simulink model "sistem_full"  (R2020b)
settings: Solver=ode45  StartTime=0.0  StopTime=10.0  MaxStep=0.01  RelTol=1e-3
undefined symbols (not defined in the file or in its folder): K_d, K_p, params, r_des
(part 1 of 2)
settings Model: Creator=Danil  LastModifiedBy=Danil

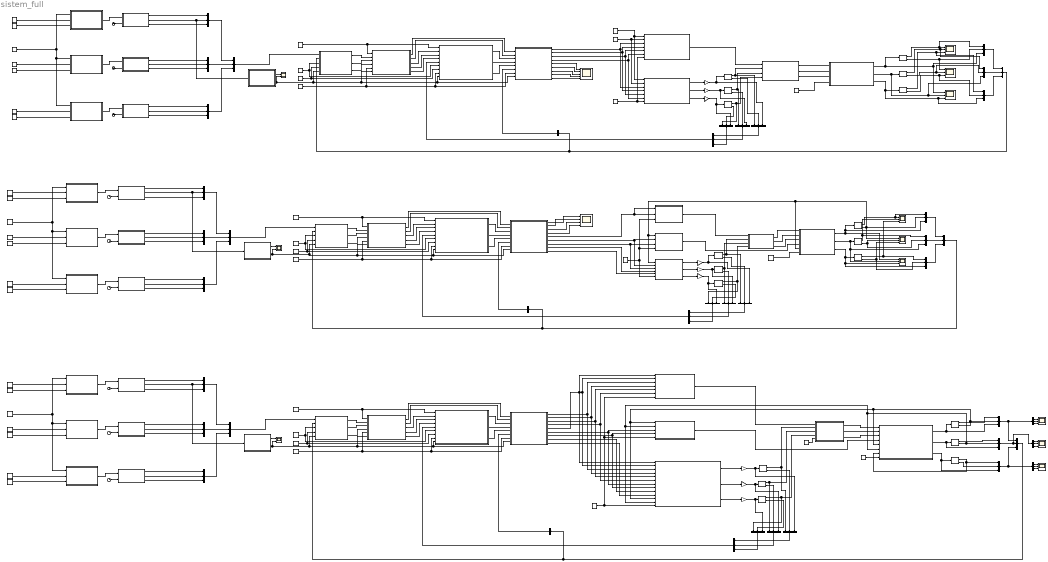
== system sistem_full ==
  note: Координаты X
  note: Траектория движения по оси X
  note: Траектория движения по оси Z
  note: Координаты Z
  note: Траектория движения по оси Y
  note: Координаты Y
  note: Траектория движения по оси Z
  note: Координаты Z
  note: Траектория движения по оси X
  note: Координаты X
  note: Траектория движения по оси Y
  note: Координаты Y
  note: Координаты X
  note: Траектория движения по оси Z
  note: Траектория движения по оси Y
  note: Траектория движения по оси X
  note: Координаты Z
  note: Координаты Y
  Bus Creator{,1..35} (36 alike) : BusCreator  Inputs=3
  Bus Selector : BusSelector  OutputSignals=x.x_dot
  Bus Selector1 : BusSelector  OutputSignals=x.x_dot
  Bus Selector2 : BusSelector  OutputSignals=x,x_dot,x_ddot
  Bus Selector3 : BusSelector  OutputSignals=y,y_dot,y_ddot
  Bus Selector4 : BusSelector  OutputSignals=z,z_dot,z_ddot
  Bus Selector5 : BusSelector  OutputSignals=x.x_dot
  Chart : Stateflow chart  TreatAsAtomicUnit=on
      settings: PortSchema="{\"entries\":[{\"content\":{\"sides\":[{\"content\":{\"connectorIds\":[\"In1\"]},\"type\":\"ConnectorPlacement.EquallySpacedRectSide\",\"uuid\":\"990aaa4d-e872-427e-8bc8-a44f7de52f17\"},{\"content\":{\"connectorIds\":[\"Out2\",\"Out1\"],\"side\":\"RIGHT\"},\"type\":\"ConnectorPlacement.EquallySpacedRectSide\",\"uuid\":\"6e7ad4a8-1d47-4f26-af3c-4dfef899b5bc\"},{\"content\":{\"connectorIds\":[],\"side\":\"TOP\"},\"type\":\"ConnectorPlacement.EquallySpacedRectSide\",\"uuid\":\"20d3b10c-4783-40ca-8243-63709ccaf162\"},{\"content\":{\"connectorIds\":[],\"side\":\"HIDDEN\"},\"type\":\"ConnectorPlacement.EquallySpacedRectSide\",\"uuid\":\"c78cf433-ac9b-47b8-aa1e-24a5718d794b\"}]},\"type\":\"ConnectorPlacement.EquallySpacedConnector\",\"uuid\":\"eb598262-5703-4057-871f-faa738de211a\"}],\"packageUris\":[\"http://schema.mathworks.com/mf0/Connector/R2020b\"],\"version\":\"1.0\"}"
  Chart1 : Stateflow chart  TreatAsAtomicUnit=on
      settings: PortSchema="{\"entries\":[{\"content\":{\"sides\":[{\"content\":{\"connectorIds\":[\"In1\"]},\"type\":\"ConnectorPlacement.EquallySpacedRectSide\",\"uuid\":\"990aaa4d-e872-427e-8bc8-a44f7de52f17\"},{\"content\":{\"connectorIds\":[\"Out2\",\"Out1\"],\"side\":\"RIGHT\"},\"type\":\"ConnectorPlacement.EquallySpacedRectSide\",\"uuid\":\"6e7ad4a8-1d47-4f26-af3c-4dfef899b5bc\"},{\"content\":{\"connectorIds\":[],\"side\":\"TOP\"},\"type\":\"ConnectorPlacement.EquallySpacedRectSide\",\"uuid\":\"20d3b10c-4783-40ca-8243-63709ccaf162\"},{\"content\":{\"connectorIds\":[],\"side\":\"HIDDEN\"},\"type\":\"ConnectorPlacement.EquallySpacedRectSide\",\"uuid\":\"c78cf433-ac9b-47b8-aa1e-24a5718d794b\"}]},\"type\":\"ConnectorPlacement.EquallySpacedConnector\",\"uuid\":\"eb598262-5703-4057-871f-faa738de211a\"}],\"packageUris\":[\"http://schema.mathworks.com/mf0/Connector/R2020b\"],\"version\":\"1.0\"}"
  Chart2 : Stateflow chart  TreatAsAtomicUnit=on
      settings: PortSchema="{\"entries\":[{\"content\":{\"sides\":[{\"content\":{\"connectorIds\":[\"In1\"]},\"type\":\"ConnectorPlacement.EquallySpacedRectSide\",\"uuid\":\"990aaa4d-e872-427e-8bc8-a44f7de52f17\"},{\"content\":{\"connectorIds\":[\"Out2\",\"Out1\"],\"side\":\"RIGHT\"},\"type\":\"ConnectorPlacement.EquallySpacedRectSide\",\"uuid\":\"6e7ad4a8-1d47-4f26-af3c-4dfef899b5bc\"},{\"content\":{\"connectorIds\":[],\"side\":\"TOP\"},\"type\":\"ConnectorPlacement.EquallySpacedRectSide\",\"uuid\":\"20d3b10c-4783-40ca-8243-63709ccaf162\"},{\"content\":{\"connectorIds\":[],\"side\":\"HIDDEN\"},\"type\":\"ConnectorPlacement.EquallySpacedRectSide\",\"uuid\":\"c78cf433-ac9b-47b8-aa1e-24a5718d794b\"}]},\"type\":\"ConnectorPlacement.EquallySpacedConnector\",\"uuid\":\"eb598262-5703-4057-871f-faa738de211a\"}],\"packageUris\":[\"http://schema.mathworks.com/mf0/Connector/R2020b\"],\"version\":\"1.0\"}"
  Clock{,1..8} (9 alike) : Clock
  Constant{,10,13,23..24,26,36} (7 alike) : Constant  Value=params  OutDataTypeStr=Bus: params_bus
  Constant1 : Constant  Value=r_des.x_0
  Constant11 : Constant  Value=0
  Constant12 : Constant  Value=r_des  OutDataTypeStr=Bus: r_des_bus
  Constant14 : Constant  Value=r_des  OutDataTypeStr=Bus: r_des_bus
  Constant15 : Constant  Value=200
  Constant16 : Constant  Value=r_des.time
  Constant17 : Constant  Value=0
  Constant{2,5,18,20} (4 alike) : Constant  Value=2
  Constant19 : Constant  Value=0
  Constant21 : Constant  Value=K_p  OutDataTypeStr=Bus: K_p_bus
  Constant22 : Constant  Value=K_d  OutDataTypeStr=Bus: K_d_bus
  Constant25 : Constant  Value=r_des.x_0
  Constant27 : Constant  Value=r_des  OutDataTypeStr=Bus: r_des_bus
  Constant28 : Constant  Value=r_des.x
  Constant29 : Constant  Value=r_des.time
  Constant3 : Constant  Value=r_des.time
  Constant30 : Constant  Value=r_des.y_0
  Constant31 : Constant  Value=r_des.y
  Constant32 : Constant  Value=r_des.z_0
  Constant33 : Constant  Value=r_des.z
  Constant34 : Constant  Value=K_p  OutDataTypeStr=Bus: K_p_bus
  Constant35 : Constant  Value=K_d  OutDataTypeStr=Bus: K_d_bus
  Constant4 : Constant  Value=r_des.y_0
  Constant6 : Constant  Value=r_des.z_0
  Constant7 : Constant  Value=10
  Constant8 : Constant  Value=K_p  OutDataTypeStr=Bus: K_p_bus
  Constant9 : Constant  Value=K_d  OutDataTypeStr=Bus: K_d_bus
  Gain : Gain  Gain=params.hor.L_x / params.hor.J_xx
  Gain1 : Gain  Gain=params.hor.L_y / params.hor.J_yy
  Gain2 : Gain  Gain=params.hor.L_z / params.hor.J_zz
  Gain3 : Gain  Gain=params.ver.L_x/params.ver.J_xx
  Gain4 : Gain  Gain=params.ver.L_y/params.ver.J_yy
  Gain5 : Gain  Gain=params.ver.L_z/params.ver.J_zz
  Gain6 : Gain  Gain=params.L_x / params.J_xx
  Gain7 : Gain  Gain=params.L_y / params.J_yy
  Gain8 : Gain  Gain=params.L_z / params.J_zz
  Integrator, Second-Order{,1..8,10..17} (17 alike) : SecondOrderIntegrator
  "Integrator, Second-Order9" : SecondOrderIntegrator  ICDXDT=14.1
  MATLAB Function : MATLAB Function  TreatAsAtomicUnit=on
  MATLAB Function1 : MATLAB Function  TreatAsAtomicUnit=on
  MATLAB Function10 : MATLAB Function  TreatAsAtomicUnit=on
  MATLAB Function11 : MATLAB Function  TreatAsAtomicUnit=on
  MATLAB Function12 : MATLAB Function  TreatAsAtomicUnit=on
  MATLAB Function13 : MATLAB Function  TreatAsAtomicUnit=on
  MATLAB Function14 : MATLAB Function  TreatAsAtomicUnit=on
  MATLAB Function15 : MATLAB Function  TreatAsAtomicUnit=on
  MATLAB Function16 : MATLAB Function  TreatAsAtomicUnit=on
  MATLAB Function17 : MATLAB Function  TreatAsAtomicUnit=on
  MATLAB Function18 : MATLAB Function  TreatAsAtomicUnit=on
  MATLAB Function19 : MATLAB Function  TreatAsAtomicUnit=on
  MATLAB Function2 : MATLAB Function  TreatAsAtomicUnit=on
  MATLAB Function20 : MATLAB Function  TreatAsAtomicUnit=on
  MATLAB Function21 : MATLAB Function  TreatAsAtomicUnit=on
  MATLAB Function22 : MATLAB Function  TreatAsAtomicUnit=on
  MATLAB Function23 : MATLAB Function  TreatAsAtomicUnit=on
  MATLAB Function24 : MATLAB Function  TreatAsAtomicUnit=on
  MATLAB Function25 : MATLAB Function  TreatAsAtomicUnit=on
  MATLAB Function26 : MATLAB Function  TreatAsAtomicUnit=on
  MATLAB Function27 : MATLAB Function  TreatAsAtomicUnit=on
  MATLAB Function28 : MATLAB Function  TreatAsAtomicUnit=on
  MATLAB Function29 : MATLAB Function  TreatAsAtomicUnit=on
  MATLAB Function3 : MATLAB Function  TreatAsAtomicUnit=on
  MATLAB Function30 : MATLAB Function  TreatAsAtomicUnit=on
  MATLAB Function31 : MATLAB Function  TreatAsAtomicUnit=on
  MATLAB Function32 : MATLAB Function  TreatAsAtomicUnit=on
  MATLAB Function33 : MATLAB Function  TreatAsAtomicUnit=on
  MATLAB Function34 : MATLAB Function  TreatAsAtomicUnit=on
  MATLAB Function35 : MATLAB Function  TreatAsAtomicUnit=on
  MATLAB Function36 : MATLAB Function  TreatAsAtomicUnit=on
  MATLAB Function37 : MATLAB Function  TreatAsAtomicUnit=on
  MATLAB Function4 : MATLAB Function  TreatAsAtomicUnit=on
  MATLAB Function5 : MATLAB Function  TreatAsAtomicUnit=on
  MATLAB Function6 : MATLAB Function  TreatAsAtomicUnit=on
  MATLAB Function7 : MATLAB Function  TreatAsAtomicUnit=on
  MATLAB Function8 : MATLAB Function  TreatAsAtomicUnit=on
  MATLAB Function9 : MATLAB Function  TreatAsAtomicUnit=on
  Scope{,1..2,5..7,11..13} (9 alike) : Scope  NumInputPorts=3
  Scope10 : Scope  NumInputPorts=2
  Scope3 : Scope  NumInputPorts=2
  Scope4 : Scope  NumInputPorts=5
  Scope8 : Scope  NumInputPorts=2
  Scope9 : Scope  NumInputPorts=4
  Subsystem : Subsystem
  Subsystem1 : Subsystem
  Subsystem2 : Subsystem
  Subsystem3 : Subsystem
  Subsystem4 : Subsystem
  Subsystem5 : Subsystem
  alpha_6 : Constant  Value=params  OutDataTypeStr=Bus: params_bus
  params : Constant  Value=params  OutDataTypeStr=Bus: params_bus
  sigma : Constant  Value=90
  w_L : Constant  Value=params.w_0
  w_R : Constant  Value=params.w_0
  wires:
  Subsystem1/2(M_y) -> MATLAB Function9/4(M_y)
  Subsystem1/3(M_z) -> MATLAB Function9/5(M_z)
  Subsystem/2(y_ddot) -> MATLAB Function7/3(y_ddot)
  Constant8/1 -> Subsystem/3(K_p), Subsystem1/6(K_p)
  Subsystem1/1(M_x) -> MATLAB Function9/3(M_x)
  Chart/1(mode) -> MATLAB Function7/6(mode), MATLAB Function9/8(mode), Subsystem1/9(mode), Subsystem/5(mode), Scope3/2
  MATLAB Function7/4(theta_des) -> Subsystem1/3(theta_des)
  Subsystem/1(x_ddot) -> MATLAB Function7/2(x_ddot)
  Constant10/1 -> MATLAB Function7/5(params), Subsystem1/8(params), MATLAB Function9/7(params)
  MATLAB Function7/1(F_T) -> MATLAB Function9/1(F_T)
  Constant9/1 -> Subsystem/4(K_d), Subsystem1/7(K_d)
  Subsystem/3(z_ddot) -> MATLAB Function7/4(z_ddot)
  MATLAB Function7/5(psi_des) -> Subsystem1/4(psi_des)
  MATLAB Function7/3(fi_des) -> Subsystem1/2(fi_des)
  MATLAB Function7/2(Y) -> MATLAB Function9/2(Y)
  Bus Creator4/1 -> Bus Creator7/1  "x"
  Bus Creator11/1 -> Subsystem1/5(r)
  Bus Creator7/1 -> Bus Selector/1, Subsystem/2(r)
  "Integrator, Second-Order"/2 -> Bus Creator8/2  "fi_dot"
  MATLAB Function11/3(M_z) -> Gain5/1
  "Integrator, Second-Order1"/2 -> Bus Creator9/2  "tehta_dot"
  Bus Creator8/1 -> Bus Creator11/1  "fi"
  "Integrator, Second-Order5"/1 -> Bus Creator6/1, Scope1/3  "z"
  Bus Creator6/1 -> Bus Creator7/3  "z"
  Bus Creator10/1 -> Bus Creator11/3  "psi"
  "Integrator, Second-Order1"/1 -> Bus Creator9/1, MATLAB Function12/3(theta)  "theta"
  Bus Creator9/1 -> Bus Creator11/2  "theta"
  MATLAB Function13/2(y_ddot) -> Bus Creator5/3, Scope2/2, "Integrator, Second-Order4"/1  "y_ddot"
  MATLAB Function9/2(alpha_2) -> MATLAB Function11/4(alpha_2), MATLAB Function10/4(alpha_2)
  "Integrator, Second-Order5"/2 -> Bus Creator6/2, Scope/3  "z_dot"
  Gain3/1 -> Bus Creator8/3, "Integrator, Second-Order"/1  "fi_ddot"
  MATLAB Function12/1(F_x) -> MATLAB Function13/1(F_x)
  MATLAB Function9/4(alpha_4) -> MATLAB Function11/6(alpha_4), MATLAB Function10/6(alpha_4)
  MATLAB Function12/3(F_z) -> MATLAB Function13/3(F_z)
  w_L/1 -> MATLAB Function10/1(w_L), MATLAB Function11/1(w_L)
  MATLAB Function10/1(F) -> MATLAB Function12/1(F)
  Gain5/1 -> "Integrator, Second-Order2"/1, Bus Creator10/3  "psi_ddot"
  alpha_6/1 -> MATLAB Function13/4(params)
  MATLAB Function9/1(alpha_1) -> MATLAB Function11/3(alpha_1), MATLAB Function10/3(alpha_1)
  params/1 -> MATLAB Function10/7(params), MATLAB Function11/7(params)
  MATLAB Function9/3(alpha_3) -> MATLAB Function11/5(alpha_3), MATLAB Function10/5(alpha_3)
  MATLAB Function13/1(x_ddot) -> "Integrator, Second-Order3"/1, Bus Creator4/3, Scope2/1  "x_ddot"
  "Integrator, Second-Order"/1 -> Bus Creator8/1, MATLAB Function12/2(fi)  "fi"
  "Integrator, Second-Order4"/1 -> Bus Creator5/1, Scope1/2  "y"
  "Integrator, Second-Order3"/1 -> Bus Creator4/1, Scope1/1  "x"
  MATLAB Function13/3(z_ddot) -> Bus Creator6/3, Scope2/3, "Integrator, Second-Order5"/1  "z_ddot"
  Gain4/1 -> Bus Creator9/3, "Integrator, Second-Order1"/1  "theta_ddot"
  MATLAB Function11/1(M_x) -> Gain3/1
  "Integrator, Second-Order2"/1 -> Bus Creator10/1, MATLAB Function12/4(psi)  "psi"
  "Integrator, Second-Order4"/2 -> Bus Creator5/2, Scope/2  "y_dot"
  MATLAB Function11/2(M_y) -> Gain4/1
  Bus Creator5/1 -> Bus Creator7/2  "y"
  "Integrator, Second-Order2"/2 -> Bus Creator10/2  "psi_dot"
  MATLAB Function12/2(F_y) -> MATLAB Function13/2(F_y)
  w_R/1 -> MATLAB Function11/2(w_R), MATLAB Function10/2(w_R)
  "Integrator, Second-Order3"/2 -> Bus Creator4/2, Scope/1  "x_dot"
  Constant2/1 -> MATLAB Function5/3(r_end)
  Bus Creator/1 -> Bus Creator3/1  "r_x"
  Bus Creator2/1 -> Bus Creator3/3  "r_z"
  MATLAB Function4/2(vel) -> Chart/1(x_dot_des), Bus Creator/2  "x_dot"
  MATLAB Function2/2(vel) -> Bus Creator2/2  "z_dot"
  Constant7/1 -> MATLAB Function3/3(r_end)
  MATLAB Function/2(vel) -> Bus Creator1/2  "y_dot"
  MATLAB Function/1(pos) -> Bus Creator1/1  "y"
  MATLAB Function1/1(coeff) -> MATLAB Function/1(coeff)
  MATLAB Function2/1(pos) -> Bus Creator2/1  "z"
  Constant6/1 -> MATLAB Function3/2(r_0)
  Constant4/1 -> MATLAB Function1/2(r_0)
  Clock1/1 -> MATLAB Function2/2(clock)
  MATLAB Function3/1(coeff) -> MATLAB Function2/1(coeff)
  Constant3/1 -> MATLAB Function3/1(t), MATLAB Function1/1(t), MATLAB Function5/1(t)
  MATLAB Function5/1(coeff) -> MATLAB Function4/1(coeff)
  Clock/1 -> MATLAB Function/2(clock)
  MATLAB Function4/3(acc) -> Bus Creator/3  "x_ddot"
  Constant5/1 -> MATLAB Function1/3(r_end)
  Constant1/1 -> MATLAB Function5/2(r_0)
  Bus Creator1/1 -> Bus Creator3/2  "r_y"
  MATLAB Function/3(acc) -> Bus Creator1/3  "y_ddot"
  MATLAB Function2/3(acc) -> Bus Creator2/3  "z_ddot"
  Clock2/1 -> MATLAB Function4/2(clock)
  MATLAB Function4/1(pos) -> Bus Creator/1  "x"
  Chart/2(sigma) -> Scope3/1
  MATLAB Function9/9(alpha_F) -> Scope4/5
  MATLAB Function9/5(w) -> Scope4/1
  MATLAB Function9/6(alpha_L) -> Scope4/2
  MATLAB Function9/7(alpha_R) -> Scope4/3
  MATLAB Function9/8(alpha_H) -> Scope4/4
  Bus Selector/1 -> MATLAB Function9/6(x_dot)  "<x_dot>"
  Bus Creator3/1 -> Subsystem/1(r_des)
  Constant12/1 -> MATLAB Function7/1(r_des), Subsystem1/1(r_des)
  Chart1/1(mode) -> MATLAB Function22/6(mode), MATLAB Function23/8(mode), Subsystem3/9(mode), Subsystem2/5(mode), Scope8/2
  Bus Creator17/1 -> Subsystem2/1(r_des)
  MATLAB Function22/2(Y) -> MATLAB Function23/2(Y)
  Clock3/1 -> MATLAB Function6/2(clock)
  MATLAB Function18/3(acc) -> Bus Creator16/3  "z_ddot"
  Clock5/1 -> MATLAB Function20/2(clock)
  MATLAB Function20/3(acc) -> Bus Creator12/3  "x_ddot"
  Subsystem2/1(x_ddot) -> MATLAB Function22/2(x_ddot)
  Chart1/2(sigma) -> Scope8/1
  Subsystem3/3(M_z) -> MATLAB Function23/5(M_z)
  MATLAB Function22/5(psi_des) -> Subsystem3/4(psi_des)
  Constant14/1 -> MATLAB Function22/1(r_des), Subsystem3/1(r_des)
  Constant17/1 -> MATLAB Function8/2(r_0)
  MATLAB Function20/2(vel) -> Chart1/1(x_dot_des), Bus Creator12/2  "x_dot"
  Bus Creator13/1 -> Bus Creator17/2  "r_y"
  Subsystem3/2(M_y) -> MATLAB Function23/4(M_y)
  Constant20/1 -> MATLAB Function19/3(r_end)
  MATLAB Function6/3(acc) -> Bus Creator13/3  "y_ddot"
  Constant16/1 -> MATLAB Function19/1(t), MATLAB Function8/1(t), MATLAB Function21/1(t)
  MATLAB Function20/1(pos) -> Bus Creator12/1  "x"
  Constant18/1 -> MATLAB Function8/3(r_end)
  MATLAB Function6/1(pos) -> Bus Creator13/1  "y"
  MATLAB Function18/2(vel) -> Bus Creator16/2  "z_dot"
  Bus Creator12/1 -> Bus Creator17/1  "r_x"
  MATLAB Function18/1(pos) -> Bus Creator16/1  "z"
  MATLAB Function19/1(coeff) -> MATLAB Function18/1(coeff)
  Constant15/1 -> MATLAB Function21/3(r_end)
  MATLAB Function6/2(vel) -> Bus Creator13/2  "y_dot"
  MATLAB Function8/1(coeff) -> MATLAB Function6/1(coeff)
  MATLAB Function21/1(coeff) -> MATLAB Function20/1(coeff)
  Constant22/1 -> Subsystem2/4(K_d), Subsystem3/7(K_d)
  Constant19/1 -> MATLAB Function19/2(r_0)
  Clock4/1 -> MATLAB Function18/2(clock)
  Subsystem2/3(z_ddot) -> MATLAB Function22/4(z_ddot)
  Bus Creator16/1 -> Bus Creator17/3  "r_z"
  MATLAB Function22/4(theta_des) -> Subsystem3/3(theta_des)
  Constant11/1 -> MATLAB Function21/2(r_0)
  MATLAB Function22/1(F_T) -> MATLAB Function23/1(F_T)
  Constant21/1 -> Subsystem2/3(K_p), Subsystem3/6(K_p)
  Subsystem3/1(M_x) -> MATLAB Function23/3(M_x)
  Constant13/1 -> MATLAB Function22/5(params), Subsystem3/8(params), MATLAB Function23/7(params)
  Subsystem2/2(y_ddot) -> MATLAB Function22/3(y_ddot)
  MATLAB Function22/3(fi_des) -> Subsystem3/2(fi_des)
  Bus Creator19/1 -> Bus Creator21/2  "y"
  MATLAB Function23/6(alpha_L) -> MATLAB Function15/2(alpha_L), MATLAB Function16/2(alpha_L)
  Bus Creator23/1 -> Bus Creator15/2  "theta"
  "Integrator, Second-Order9"/1 -> Bus Creator18/1, Scope6/1  "x"
  Bus Creator15/1 -> Subsystem3/5(r)
  MATLAB Function17/1(F_x) -> MATLAB Function24/1(F_x)
  Bus Creator20/1 -> Bus Creator21/3  "z"
  "Integrator, Second-Order8"/2 -> Bus Creator14/2  "psi_dot"
  "Integrator, Second-Order6"/2 -> Bus Creator22/2  "fi_dot"
  Gain/1 -> Bus Creator22/3, "Integrator, Second-Order6"/1  "fi_ddot"
  Bus Creator21/1 -> Bus Selector1/1, Subsystem2/2(r)
  MATLAB Function16/1(M_x) -> Gain/1
  MATLAB Function24/2(y_ddot) -> Bus Creator19/3, Scope7/2, "Integrator, Second-Order10"/1  "y_ddot"
  Constant24/1 -> MATLAB Function24/6(params)
  "Integrator, Second-Order11"/2 -> Scope5/3, Bus Creator20/2  "z_dot"
  MATLAB Function17/2(F_y) -> MATLAB Function24/2(F_y)
  "Integrator, Second-Order7"/1 -> MATLAB Function17/3(theta), Bus Creator23/1  "theta"
  "Integrator, Second-Order8"/1 -> MATLAB Function17/4(psi), Bus Creator14/1  "psi"
  "Integrator, Second-Order11"/1 -> Bus Creator20/1, Scope6/3  "z"
  MATLAB Function14/1(F) -> MATLAB Function17/1(F)
  Gain1/1 -> Bus Creator23/3, "Integrator, Second-Order7"/1  "theta_ddot"
  Gain2/1 -> Bus Creator14/3, "Integrator, Second-Order8"/1  "psi_ddot"
  "Integrator, Second-Order6"/1 -> Bus Creator22/1, MATLAB Function17/2(fi)  "fi"
  Bus Creator18/1 -> Bus Creator21/1  "x"
  MATLAB Function16/3(M_z) -> Gain2/1
  "Integrator, Second-Order10"/1 -> Bus Creator19/1, Scope6/2  "y"
  MATLAB Function23/8(alpha_H) -> MATLAB Function16/4(alpha_H)
  MATLAB Function17/3(F_z) -> MATLAB Function24/3(F_z)
  MATLAB Function24/1(x_ddot) -> Bus Creator18/3, "Integrator, Second-Order9"/1, Scope7/1  "x_ddot"
  "Integrator, Second-Order10"/2 -> Scope5/2, Bus Creator19/2  "y_dot"
  MATLAB Function23/9(alpha_F) -> MATLAB Function16/5(alpha_F)
  MATLAB Function15/1(Y) -> MATLAB Function24/4(Y)
  MATLAB Function16/2(M_y) -> Gain1/1
  MATLAB Function24/3(z_ddot) -> Bus Creator20/3, Scope7/3, "Integrator, Second-Order11"/1  "z_ddot"
  "Integrator, Second-Order9"/2 -> MATLAB Function24/5(x_dot), MATLAB Function16/1(x_dot), MATLAB Function15/1(x_dot), Bus Creator18/2, Scope5/1  "x_dot"
  Bus Creator22/1 -> Bus Creator15/1  "fi"
  MATLAB Function23/5(w) -> MATLAB Function14/1(w_L), MATLAB Function14/2(w_R)
  Constant23/1 -> MATLAB Function16/6(params), MATLAB Function14/3(params), MATLAB Function15/4(params)
  MATLAB Function23/7(alpha_R) -> MATLAB Function16/3(alpha_R), MATLAB Function15/3(alpha_R)
  "Integrator, Second-Order7"/2 -> Bus Creator23/2  "theta_dot"
  Bus Creator14/1 -> Bus Creator15/3  "psi"
  Bus Selector1/1 -> MATLAB Function23/6(x_dot)  "<x_dot>"
  MATLAB Function23/1(alpha_1) -> Scope9/1
  MATLAB Function23/2(alpha_2) -> Scope9/2
  MATLAB Function23/3(alpha_3) -> Scope9/3
  MATLAB Function23/4(alpha_4) -> Scope9/4
  MATLAB Function26/1(coeff) -> MATLAB Function25/1(coeff)
  Constant31/1 -> MATLAB Function32/3(r_end)
  MATLAB Function29/5(psi_des) -> Subsystem5/4(psi_des)
  Constant27/1 -> MATLAB Function29/1(r_des), Subsystem5/1(r_des)
  MATLAB Function27/3(acc) -> Bus Creator24/3  "x_ddot"
  Bus Creator26/1 -> Bus Creator27/3  "r_z"
  Constant35/1 -> Subsystem4/4(K_d), Subsystem5/7(K_d)
  MATLAB Function27/1(pos) -> Bus Creator24/1  "x"
  MATLAB Function29/3(fi_des) -> Subsystem5/2(fi_des)
  MATLAB Function27/2(vel) -> Chart2/1(x_dot_des), Bus Creator24/2  "x_dot"
  Constant32/1 -> MATLAB Function26/2(r_0)
  Clock7/1 -> MATLAB Function25/2(clock)
  Constant34/1 -> Subsystem4/3(K_p), Subsystem5/6(K_p)
  MATLAB Function28/1(coeff) -> MATLAB Function27/1(coeff)
  Subsystem5/1(M_x) -> MATLAB Function30/3(M_x)
  Subsystem4/2(y_ddot) -> MATLAB Function29/3(y_ddot)
  Chart2/1(mode) -> MATLAB Function29/6(mode), MATLAB Function30/8(mode), Subsystem5/9(mode), Subsystem4/5(mode), Scope10/2
  Subsystem4/1(x_ddot) -> MATLAB Function29/2(x_ddot)
  MATLAB Function29/4(theta_des) -> Subsystem5/3(theta_des)
  Constant25/1 -> MATLAB Function28/2(r_0)
  MATLAB Function29/1(F_T) -> MATLAB Function30/1(F_T)
  Subsystem4/3(z_ddot) -> MATLAB Function29/4(z_ddot)
  MATLAB Function31/1(pos) -> Bus Creator25/1  "y"
  MATLAB Function31/3(acc) -> Bus Creator25/3  "y_ddot"
  MATLAB Function31/2(vel) -> Bus Creator25/2  "y_dot"
  Constant28/1 -> MATLAB Function28/3(r_end)
  MATLAB Function25/1(pos) -> Bus Creator26/1  "z"
  Bus Creator24/1 -> Bus Creator27/1  "r_x"
  MATLAB Function32/1(coeff) -> MATLAB Function31/1(coeff)
  MATLAB Function25/2(vel) -> Bus Creator26/2  "z_dot"
  Subsystem5/3(M_z) -> MATLAB Function30/5(M_z)
  Chart2/2(sigma) -> Scope10/1
  Constant30/1 -> MATLAB Function32/2(r_0)
  Constant33/1 -> MATLAB Function26/3(r_end)
  MATLAB Function25/3(acc) -> Bus Creator26/3  "z_ddot"
  Bus Creator25/1 -> Bus Creator27/2  "r_y"
  Clock8/1 -> MATLAB Function27/2(clock)
  Bus Creator27/1 -> Subsystem4/1(r_des)
  Constant26/1 -> MATLAB Function29/5(params), Subsystem5/8(params), MATLAB Function30/7(params)
  Subsystem5/2(M_y) -> MATLAB Function30/4(M_y)
  Clock6/1 -> MATLAB Function31/2(clock)
  Constant29/1 -> MATLAB Function26/1(t), MATLAB Function32/1(t), MATLAB Function28/1(t)
  MATLAB Function29/2(Y) -> MATLAB Function30/2(Y)
  Gain6/1 -> Bus Creator34/3, "Integrator, Second-Order12"/1  "fi_ddot"
  MATLAB Function37/1(x_ddot) -> Bus Creator28/3, "Integrator, Second-Order15"/1
  MATLAB Function37/3(z_ddot) -> Bus Creator30/3, "Integrator, Second-Order17"/1
  MATLAB Function30/5(w) -> MATLAB Function35/2(w_R), MATLAB Function33/2(w_R), MATLAB Function33/1(w_L), MATLAB Function35/1(w_L)
  Gain8/1 -> Bus Creator32/3, "Integrator, Second-Order14"/1  "psi_ddot"
  MATLAB Function36/1(F_x) -> MATLAB Function37/1(F_x)
  MATLAB Function37/2(y_ddot) -> Bus Creator29/3, "Integrator, Second-Order16"/1
  MATLAB Function36/3(F_z) -> MATLAB Function37/3(F_z)
  "Integrator, Second-Order16"/2 -> MATLAB Function37/6(y_dot), MATLAB Function34/2(y_dot), MATLAB Function35/12(y_dot), Bus Creator29/2  "y_dot"
  MATLAB Function30/1(alpha_1) -> MATLAB Function35/3(alpha_1), MATLAB Function33/3(alpha_1)
  MATLAB Function30/6(alpha_L) -> MATLAB Function35/7(alpha_L), MATLAB Function34/3(alpha_L)
  MATLAB Function30/4(alpha_4) -> MATLAB Function35/6(alpha_4), MATLAB Function33/6(alpha_4)
  Gain7/1 -> Bus Creator35/3, "Integrator, Second-Order13"/1  "theta_ddot"
  "Integrator, Second-Order15"/2 -> Bus Creator28/2, MATLAB Function37/5(x_dot), MATLAB Function34/1(x_dot), MATLAB Function35/11(x_dot)  "x_dot"
  MATLAB Function34/1(Y) -> MATLAB Function37/4(Y)
  Constant/1 -> MATLAB Function35/13(params), MATLAB Function34/5(params), MATLAB Function33/7(params)
  MATLAB Function35/3(M_z) -> Gain8/1
  Constant36/1 -> MATLAB Function37/8(params)
  "Integrator, Second-Order12"/1 -> MATLAB Function36/2(fi), Bus Creator34/1  "fi"
  MATLAB Function33/1(F) -> MATLAB Function36/1(F)
  MATLAB Function30/2(alpha_2) -> MATLAB Function35/4(alpha_2), MATLAB Function33/4(alpha_2)
  MATLAB Function35/1(M_x) -> Gain6/1
  MATLAB Function30/9(alpha_F) -> MATLAB Function35/10(alpha_F)
  MATLAB Function30/8(alpha_H) -> MATLAB Function35/9(alpha_H)
  MATLAB Function36/2(F_y) -> MATLAB Function37/2(F_y)
  MATLAB Function30/7(alpha_R) -> MATLAB Function35/8(alpha_R), MATLAB Function34/4(alpha_R)
  MATLAB Function35/2(M_y) -> Gain7/1
  MATLAB Function30/3(alpha_3) -> MATLAB Function35/5(alpha_3), MATLAB Function33/5(alpha_3)
  sigma/1 -> MATLAB Function36/5(sigma)
  "Integrator, Second-Order14"/1 -> Bus Creator32/1, MATLAB Function36/4(psi)  "psi"
  "Integrator, Second-Order17"/1 -> Bus Creator30/1, MATLAB Function37/7(z_dot)  "z"
  "Integrator, Second-Order13"/1 -> MATLAB Function36/3(theta), Bus Creator35/1  "theta"
  Bus Creator28/1 -> Bus Creator31/1, Bus Selector2/1  "x"
  Bus Creator29/1 -> Bus Selector3/1, Bus Creator31/2  "y"
  Bus Creator30/1 -> Bus Selector4/1, Bus Creator31/3  "z"
  Bus Creator32/1 -> Bus Creator33/3  "psi"
  Bus Creator34/1 -> Bus Creator33/1  "fi"
  Bus Creator35/1 -> Bus Creator33/2  "theta"
  "Integrator, Second-Order15"/1 -> Bus Creator28/1  "x"
  "Integrator, Second-Order16"/1 -> Bus Creator29/1  "y"
  "Integrator, Second-Order17"/2 -> Bus Creator30/2  "z_dot"
  Bus Selector3/2 -> Scope11/2  "<y_dot>"
  Bus Selector3/3 -> Scope11/3  "<y_ddot>"
  Bus Selector3/1 -> Scope11/1  "<y>"
  Bus Selector4/2 -> Scope13/2  "<z_dot>"
  Bus Selector4/3 -> Scope13/3  "<z_ddot>"
  Bus Selector4/1 -> Scope13/1  "<z>"
  Bus Selector2/2 -> Scope12/2  "<x_dot>"
  Bus Selector2/3 -> Scope12/3  "<x_ddot>"
  Bus Selector2/1 -> Scope12/1  "<x>"
  "Integrator, Second-Order12"/2 -> Bus Creator34/2  "fi_dot"
  "Integrator, Second-Order13"/2 -> Bus Creator35/2  "theta_dot"
  "Integrator, Second-Order14"/2 -> Bus Creator32/2  "psi_dot"
  Bus Creator31/1 -> Bus Selector5/1, Subsystem4/2(r)
  Bus Creator33/1 -> Subsystem5/5(r)
  Bus Selector5/1 -> MATLAB Function30/6(x_dot)  "<x_dot>"

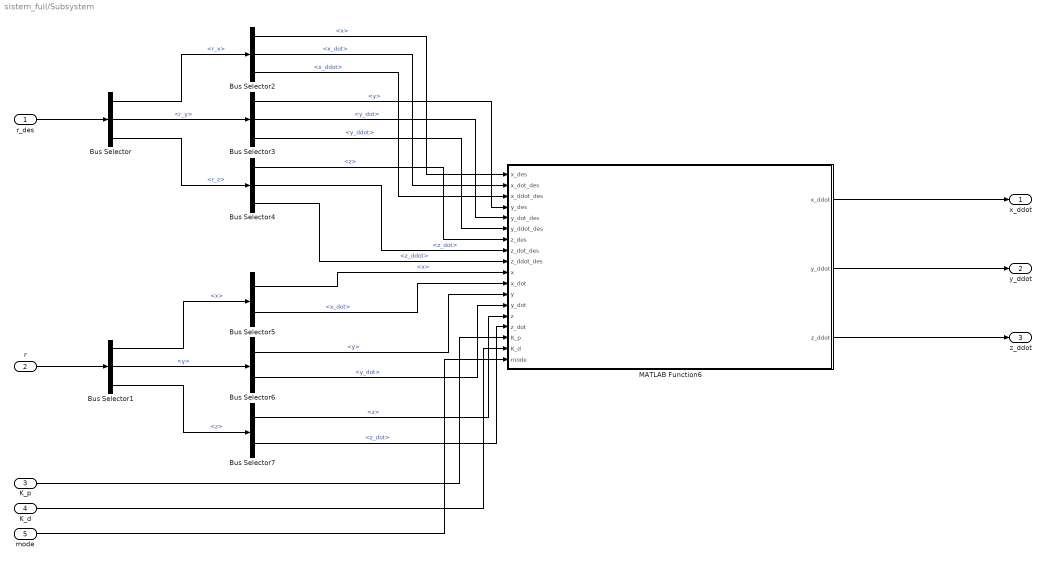
== system sistem_full/Subsystem ==
  r_des : Inport
  r : Inport  Port=2
  K_p : Inport  Port=3
  K_d : Inport  Port=4
  mode : Inport  Port=5
  Bus Selector : BusSelector  OutputSignals=r_x,r_y,r_z
  Bus Selector1 : BusSelector  OutputSignals=x,y,z
  Bus Selector2 : BusSelector  OutputSignals=x,x_dot,x_ddot
  Bus Selector3 : BusSelector  OutputSignals=y,y_dot,y_ddot
  Bus Selector4 : BusSelector  OutputSignals=z,z_dot,z_ddot
  Bus Selector5 : BusSelector  OutputSignals=x,x_dot
  Bus Selector6 : BusSelector  OutputSignals=y,y_dot
  Bus Selector7 : BusSelector  OutputSignals=z,z_dot
  MATLAB Function6 : MATLAB Function  TreatAsAtomicUnit=on
  x_ddot : Outport
  y_ddot : Outport  Port=2
  z_ddot : Outport  Port=3
  wires:
  Bus Selector3/1 -> MATLAB Function6/4(y_des)  "<y>"
  Bus Selector4/3 -> MATLAB Function6/9(z_ddot_des)  "<z_ddot>"
  Bus Selector4/1 -> MATLAB Function6/7(z_des)  "<z>"
  Bus Selector/1 -> Bus Selector2/1  "<r_x>"
  Bus Selector5/2 -> MATLAB Function6/11(x_dot)  "<x_dot>"
  Bus Selector3/2 -> MATLAB Function6/5(y_dot_des)  "<y_dot>"
  Bus Selector/3 -> Bus Selector4/1  "<r_z>"
  r/1 -> Bus Selector1/1
  r_des/1 -> Bus Selector/1
  Bus Selector2/1 -> MATLAB Function6/1(x_des)  "<x>"
  Bus Selector5/1 -> MATLAB Function6/10(x)  "<x>"
  MATLAB Function6/2(y_ddot) -> y_ddot/1
  MATLAB Function6/3(z_ddot) -> z_ddot/1
  K_d/1 -> MATLAB Function6/17(K_d)
  K_p/1 -> MATLAB Function6/16(K_p)
  Bus Selector1/3 -> Bus Selector7/1  "<z>"
  Bus Selector2/2 -> MATLAB Function6/2(x_dot_des)  "<x_dot>"
  Bus Selector7/2 -> MATLAB Function6/15(z_dot)  "<z_dot>"
  MATLAB Function6/1(x_ddot) -> x_ddot/1
  Bus Selector6/1 -> MATLAB Function6/12(y)  "<y>"
  Bus Selector7/1 -> MATLAB Function6/14(z)  "<z>"
  Bus Selector4/2 -> MATLAB Function6/8(z_dot_des)  "<z_dot>"
  Bus Selector2/3 -> MATLAB Function6/3(x_ddot_des)  "<x_ddot>"
  Bus Selector1/1 -> Bus Selector5/1  "<x>"
  Bus Selector1/2 -> Bus Selector6/1  "<y>"
  Bus Selector6/2 -> MATLAB Function6/13(y_dot)  "<y_dot>"
  Bus Selector3/3 -> MATLAB Function6/6(y_ddot_des)  "<y_ddot>"
  Bus Selector/2 -> Bus Selector3/1  "<r_y>"
  mode/1 -> MATLAB Function6/18(mode)

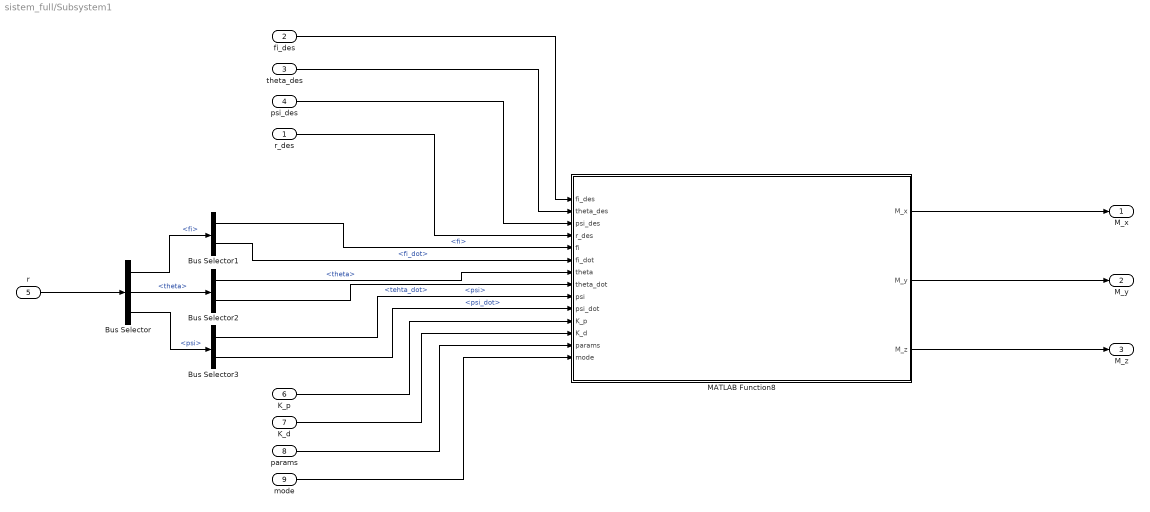
== system sistem_full/Subsystem1 ==
  r_des : Inport
  fi_des : Inport  Port=2
  theta_des : Inport  Port=3
  psi_des : Inport  Port=4
  r : Inport  Port=5
  K_p : Inport  Port=6
  K_d : Inport  Port=7
  params : Inport  Port=8
  mode : Inport  Port=9
  Bus Selector : BusSelector  OutputSignals=fi,theta,psi
  Bus Selector1 : BusSelector  OutputSignals=fi,fi_dot
  Bus Selector2 : BusSelector  OutputSignals=theta,tehta_dot
  Bus Selector3 : BusSelector  OutputSignals=psi,psi_dot
  MATLAB Function8 : MATLAB Function  TreatAsAtomicUnit=on
  M_x : Outport
  M_y : Outport  Port=2
  M_z : Outport  Port=3
  wires:
  Bus Selector3/1 -> MATLAB Function8/9(psi)  "<psi>"
  Bus Selector1/2 -> MATLAB Function8/6(fi_dot)  "<fi_dot>"
  Bus Selector/1 -> Bus Selector1/1  "<fi>"
  Bus Selector1/1 -> MATLAB Function8/5(fi)  "<fi>"
  r/1 -> Bus Selector/1
  MATLAB Function8/3(M_z) -> M_z/1
  MATLAB Function8/1(M_x) -> M_x/1
  MATLAB Function8/2(M_y) -> M_y/1
  Bus Selector2/2 -> MATLAB Function8/8(theta_dot)  "<tehta_dot>"
  K_p/1 -> MATLAB Function8/11(K_p)
  Bus Selector2/1 -> MATLAB Function8/7(theta)  "<theta>"
  Bus Selector/2 -> Bus Selector2/1  "<theta>"
  r_des/1 -> MATLAB Function8/4(r_des)
  params/1 -> MATLAB Function8/13(params)
  psi_des/1 -> MATLAB Function8/3(psi_des)
  fi_des/1 -> MATLAB Function8/1(fi_des)
  K_d/1 -> MATLAB Function8/12(K_d)
  theta_des/1 -> MATLAB Function8/2(theta_des)
  Bus Selector3/2 -> MATLAB Function8/10(psi_dot)  "<psi_dot>"
  Bus Selector/3 -> Bus Selector3/1  "<psi>"
  mode/1 -> MATLAB Function8/14(mode)

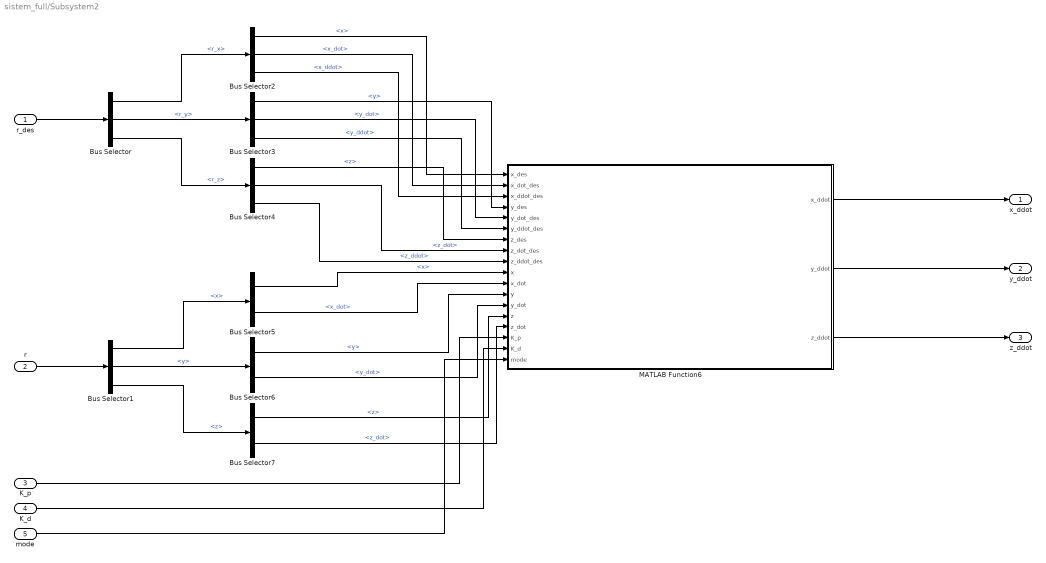
== system sistem_full/Subsystem2 ==
  r_des : Inport
  r : Inport  Port=2
  K_p : Inport  Port=3
  K_d : Inport  Port=4
  mode : Inport  Port=5
  Bus Selector : BusSelector  OutputSignals=r_x,r_y,r_z
  Bus Selector1 : BusSelector  OutputSignals=x,y,z
  Bus Selector2 : BusSelector  OutputSignals=x,x_dot,x_ddot
  Bus Selector3 : BusSelector  OutputSignals=y,y_dot,y_ddot
  Bus Selector4 : BusSelector  OutputSignals=z,z_dot,z_ddot
  Bus Selector5 : BusSelector  OutputSignals=x,x_dot
  Bus Selector6 : BusSelector  OutputSignals=y,y_dot
  Bus Selector7 : BusSelector  OutputSignals=z,z_dot
  MATLAB Function6 : MATLAB Function  TreatAsAtomicUnit=on
  x_ddot : Outport
  y_ddot : Outport  Port=2
  z_ddot : Outport  Port=3
  wires:
  Bus Selector3/1 -> MATLAB Function6/4(y_des)  "<y>"
  Bus Selector4/3 -> MATLAB Function6/9(z_ddot_des)  "<z_ddot>"
  Bus Selector4/1 -> MATLAB Function6/7(z_des)  "<z>"
  Bus Selector/1 -> Bus Selector2/1  "<r_x>"
  Bus Selector5/2 -> MATLAB Function6/11(x_dot)  "<x_dot>"
  Bus Selector3/2 -> MATLAB Function6/5(y_dot_des)  "<y_dot>"
  Bus Selector/3 -> Bus Selector4/1  "<r_z>"
  r/1 -> Bus Selector1/1
  r_des/1 -> Bus Selector/1
  Bus Selector2/1 -> MATLAB Function6/1(x_des)  "<x>"
  Bus Selector5/1 -> MATLAB Function6/10(x)  "<x>"
  MATLAB Function6/2(y_ddot) -> y_ddot/1
  MATLAB Function6/3(z_ddot) -> z_ddot/1
  K_d/1 -> MATLAB Function6/17(K_d)
  K_p/1 -> MATLAB Function6/16(K_p)
  Bus Selector1/3 -> Bus Selector7/1  "<z>"
  Bus Selector2/2 -> MATLAB Function6/2(x_dot_des)  "<x_dot>"
  Bus Selector7/2 -> MATLAB Function6/15(z_dot)  "<z_dot>"
  MATLAB Function6/1(x_ddot) -> x_ddot/1
  Bus Selector6/1 -> MATLAB Function6/12(y)  "<y>"
  Bus Selector7/1 -> MATLAB Function6/14(z)  "<z>"
  Bus Selector4/2 -> MATLAB Function6/8(z_dot_des)  "<z_dot>"
  Bus Selector2/3 -> MATLAB Function6/3(x_ddot_des)  "<x_ddot>"
  Bus Selector1/1 -> Bus Selector5/1  "<x>"
  Bus Selector1/2 -> Bus Selector6/1  "<y>"
  Bus Selector6/2 -> MATLAB Function6/13(y_dot)  "<y_dot>"
  Bus Selector3/3 -> MATLAB Function6/6(y_ddot_des)  "<y_ddot>"
  Bus Selector/2 -> Bus Selector3/1  "<r_y>"
  mode/1 -> MATLAB Function6/18(mode)

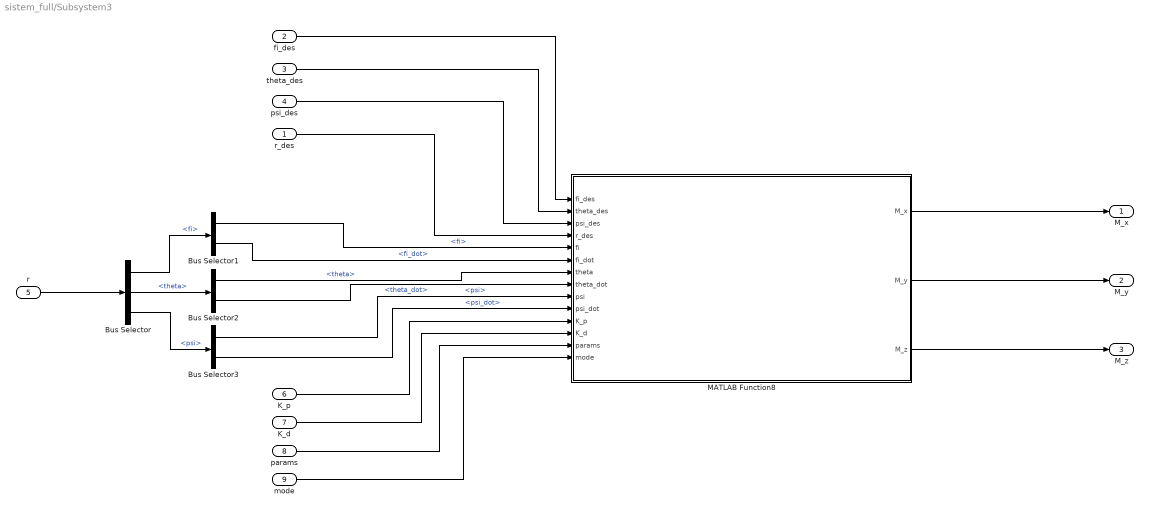
== system sistem_full/Subsystem3 ==
  r_des : Inport
  fi_des : Inport  Port=2
  theta_des : Inport  Port=3
  psi_des : Inport  Port=4
  r : Inport  Port=5
  K_p : Inport  Port=6
  K_d : Inport  Port=7
  params : Inport  Port=8
  mode : Inport  Port=9
  Bus Selector : BusSelector  OutputSignals=fi,theta,psi
  Bus Selector1 : BusSelector  OutputSignals=fi,fi_dot
  Bus Selector2 : BusSelector  OutputSignals=theta,theta_dot
  Bus Selector3 : BusSelector  OutputSignals=psi,psi_dot
  MATLAB Function8 : MATLAB Function  TreatAsAtomicUnit=on
  M_x : Outport
  M_y : Outport  Port=2
  M_z : Outport  Port=3
  wires:
  Bus Selector3/1 -> MATLAB Function8/9(psi)  "<psi>"
  Bus Selector1/2 -> MATLAB Function8/6(fi_dot)  "<fi_dot>"
  Bus Selector/1 -> Bus Selector1/1  "<fi>"
  Bus Selector1/1 -> MATLAB Function8/5(fi)  "<fi>"
  r/1 -> Bus Selector/1
  MATLAB Function8/3(M_z) -> M_z/1
  MATLAB Function8/1(M_x) -> M_x/1
  MATLAB Function8/2(M_y) -> M_y/1
  Bus Selector2/2 -> MATLAB Function8/8(theta_dot)  "<theta_dot>"
  K_p/1 -> MATLAB Function8/11(K_p)
  Bus Selector2/1 -> MATLAB Function8/7(theta)  "<theta>"
  Bus Selector/2 -> Bus Selector2/1  "<theta>"
  r_des/1 -> MATLAB Function8/4(r_des)
  params/1 -> MATLAB Function8/13(params)
  psi_des/1 -> MATLAB Function8/3(psi_des)
  fi_des/1 -> MATLAB Function8/1(fi_des)
  K_d/1 -> MATLAB Function8/12(K_d)
  theta_des/1 -> MATLAB Function8/2(theta_des)
  Bus Selector3/2 -> MATLAB Function8/10(psi_dot)  "<psi_dot>"
  Bus Selector/3 -> Bus Selector3/1  "<psi>"
  mode/1 -> MATLAB Function8/14(mode)

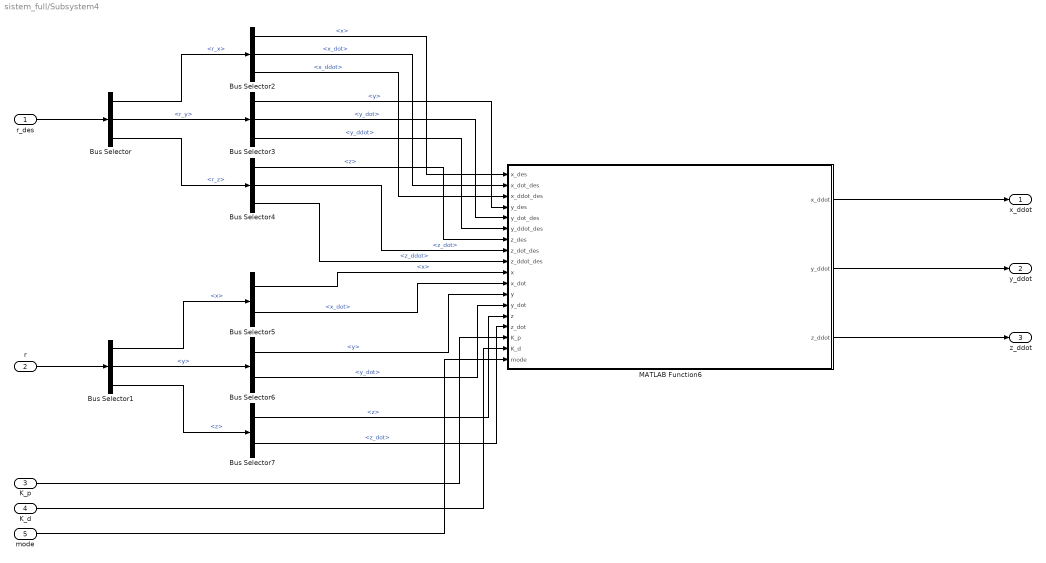
== system sistem_full/Subsystem4 ==
  r_des : Inport
  r : Inport  Port=2
  K_p : Inport  Port=3
  K_d : Inport  Port=4
  mode : Inport  Port=5
  Bus Selector : BusSelector  OutputSignals=r_x,r_y,r_z
  Bus Selector1 : BusSelector  OutputSignals=x,y,z
  Bus Selector2 : BusSelector  OutputSignals=x,x_dot,x_ddot
  Bus Selector3 : BusSelector  OutputSignals=y,y_dot,y_ddot
  Bus Selector4 : BusSelector  OutputSignals=z,z_dot,z_ddot
  Bus Selector5 : BusSelector  OutputSignals=x,x_dot
  Bus Selector6 : BusSelector  OutputSignals=y,y_dot
  Bus Selector7 : BusSelector  OutputSignals=z,z_dot
  MATLAB Function6 : MATLAB Function  TreatAsAtomicUnit=on
  x_ddot : Outport
  y_ddot : Outport  Port=2
  z_ddot : Outport  Port=3
  wires:
  Bus Selector3/1 -> MATLAB Function6/4(y_des)  "<y>"
  Bus Selector4/3 -> MATLAB Function6/9(z_ddot_des)  "<z_ddot>"
  Bus Selector4/1 -> MATLAB Function6/7(z_des)  "<z>"
  Bus Selector/1 -> Bus Selector2/1  "<r_x>"
  Bus Selector5/2 -> MATLAB Function6/11(x_dot)  "<x_dot>"
  Bus Selector3/2 -> MATLAB Function6/5(y_dot_des)  "<y_dot>"
  Bus Selector/3 -> Bus Selector4/1  "<r_z>"
  r/1 -> Bus Selector1/1
  r_des/1 -> Bus Selector/1
  Bus Selector2/1 -> MATLAB Function6/1(x_des)  "<x>"
  Bus Selector5/1 -> MATLAB Function6/10(x)  "<x>"
  MATLAB Function6/2(y_ddot) -> y_ddot/1
  MATLAB Function6/3(z_ddot) -> z_ddot/1
  K_d/1 -> MATLAB Function6/17(K_d)
  K_p/1 -> MATLAB Function6/16(K_p)
  Bus Selector1/3 -> Bus Selector7/1  "<z>"
  Bus Selector2/2 -> MATLAB Function6/2(x_dot_des)  "<x_dot>"
  Bus Selector7/2 -> MATLAB Function6/15(z_dot)  "<z_dot>"
  MATLAB Function6/1(x_ddot) -> x_ddot/1
  Bus Selector6/1 -> MATLAB Function6/12(y)  "<y>"
  Bus Selector7/1 -> MATLAB Function6/14(z)  "<z>"
  Bus Selector4/2 -> MATLAB Function6/8(z_dot_des)  "<z_dot>"
  Bus Selector2/3 -> MATLAB Function6/3(x_ddot_des)  "<x_ddot>"
  Bus Selector1/1 -> Bus Selector5/1  "<x>"
  Bus Selector1/2 -> Bus Selector6/1  "<y>"
  Bus Selector6/2 -> MATLAB Function6/13(y_dot)  "<y_dot>"
  Bus Selector3/3 -> MATLAB Function6/6(y_ddot_des)  "<y_ddot>"
  Bus Selector/2 -> Bus Selector3/1  "<r_y>"
  mode/1 -> MATLAB Function6/18(mode)

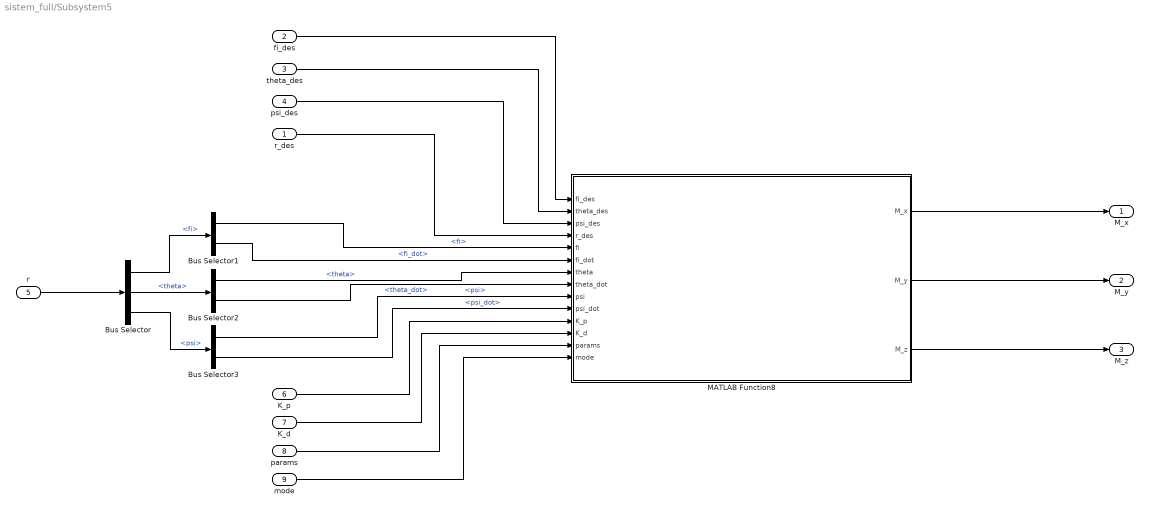
== system sistem_full/Subsystem5 ==
  r_des : Inport
  fi_des : Inport  Port=2
  theta_des : Inport  Port=3
  psi_des : Inport  Port=4
  r : Inport  Port=5
  K_p : Inport  Port=6
  K_d : Inport  Port=7
  params : Inport  Port=8
  mode : Inport  Port=9
  Bus Selector : BusSelector  OutputSignals=fi,theta,psi
  Bus Selector1 : BusSelector  OutputSignals=fi,fi_dot
  Bus Selector2 : BusSelector  OutputSignals=theta,theta_dot
  Bus Selector3 : BusSelector  OutputSignals=psi,psi_dot
  MATLAB Function8 : MATLAB Function  TreatAsAtomicUnit=on
  M_x : Outport
  M_y : Outport  Port=2
  M_z : Outport  Port=3
  wires:
  Bus Selector3/1 -> MATLAB Function8/9(psi)  "<psi>"
  Bus Selector1/2 -> MATLAB Function8/6(fi_dot)  "<fi_dot>"
  Bus Selector/1 -> Bus Selector1/1  "<fi>"
  Bus Selector1/1 -> MATLAB Function8/5(fi)  "<fi>"
  r/1 -> Bus Selector/1
  MATLAB Function8/3(M_z) -> M_z/1
  MATLAB Function8/1(M_x) -> M_x/1
  MATLAB Function8/2(M_y) -> M_y/1
  Bus Selector2/2 -> MATLAB Function8/8(theta_dot)  "<theta_dot>"
  K_p/1 -> MATLAB Function8/11(K_p)
  Bus Selector2/1 -> MATLAB Function8/7(theta)  "<theta>"
  Bus Selector/2 -> Bus Selector2/1  "<theta>"
  r_des/1 -> MATLAB Function8/4(r_des)
  params/1 -> MATLAB Function8/13(params)
  psi_des/1 -> MATLAB Function8/3(psi_des)
  fi_des/1 -> MATLAB Function8/1(fi_des)
  K_d/1 -> MATLAB Function8/12(K_d)
  theta_des/1 -> MATLAB Function8/2(theta_des)
  Bus Selector3/2 -> MATLAB Function8/10(psi_dot)  "<psi_dot>"
  Bus Selector/3 -> Bus Selector3/1  "<psi>"
  mode/1 -> MATLAB Function8/14(mode)

== matlab function sistem_full/MATLAB Function7 ==
  data: r_des input; F_T output; Y output; fi_des output; x_ddot input; y_ddot input; z_ddot input; params input; mode input; theta_des output; psi_des output
function [F_T, Y, fi_des, theta_des, psi_des] = fcn(r_des, x_ddot, y_ddot, z_ddot, params, mode)

if mode == 0
    
    F_T = params.m * (z_ddot + params.g);
    Y = 0;

    fi_des = (1 / params.g) * (x_ddot * sin(r_des.psi) - y_ddot * cos(r_des.psi));
    theta_des = (1 / params.g) * (x_ddot * cos(r_des.psi) + y_ddot * sin(r_des.psi));
    psi_des = r_des.psi;
    
elseif mode == 1
    
    %F_T = params.m * x_ddot + params.k_x * x_dot;

    F_T = params.m * x_ddot + r_des.x_dot;
    Y = params.m * params.g;

    fi_des = r_des.fi;
    theta_des = (params.m / (params.k_x * r_des.x_dot)) * (y_ddot * sin(r_des.fi) - z_ddot * cos(r_des.fi));
    psi_des = (params.m / (params.k_x * r_des.x_dot)) * (y_ddot * cos(r_des.fi) + z_ddot * sin(r_des.fi));

    %theta_des = (params.m / F_T) * (y_ddot * sin(r_des.fi) - z_ddot * cos(r_des.fi));
    %psi_des = (params.m / F_T) * (y_ddot * cos(r_des.fi) + z_ddot * sin(r_des.fi));
    
else 
    
    F_T = params.m * (z_ddot + params.g);
    Y = 0;

    fi_des = (1 / params.g) * (x_ddot * sin(r_des.psi) - y_ddot * cos(r_des.psi));
    theta_des = (1 / params.g) * (x_ddot * cos(r_des.psi) + y_ddot * sin(r_des.psi));
    psi_des = r_des.psi;
    
end

== matlab function sistem_full/Subsystem1/MATLAB Function8 ==
  data: fi_des input; theta_des input; psi_des input; r_des input; fi input; fi_dot input; theta input; theta_dot input; psi input; psi_dot input; M_x output; K_p input; K_d input; params input; M_y output; M_z output; mode input
function [M_x, M_y, M_z] = fcn(fi_des, theta_des, psi_des, r_des, fi, fi_dot, theta, theta_dot, psi, psi_dot, K_p, K_d, params, mode)

if mode == 0

    M_x = (params.ver.J_xx / params.ver.L_x) * (r_des.fi_ddot + abs(K_d.ver.fi) * (r_des.fi_dot - fi_dot) + abs(K_p.ver.fi) * (fi_des - fi));
    M_y = (params.ver.J_yy / params.ver.L_y) * (r_des.theta_ddot + abs(K_d.ver.theta) * (r_des.theta_dot - theta_dot) + abs(K_p.ver.theta) * (theta_des - theta));
    M_z = (params.ver.J_zz / params.ver.L_z) * (r_des.psi_ddot + abs(K_d.ver.psi) * (r_des.psi_dot - psi_dot) + abs(K_p.ver.psi) * (psi_des - psi));
    
elseif mode == 1
    
    M_x = (params.hor.J_xx / params.hor.L_x) * (r_des.fi_ddot + abs(K_d.hor.fi) * (r_des.fi_dot - fi_dot) + abs(K_p.hor.fi) * (fi_des - fi));
    M_y = (params.hor.J_yy / params.hor.L_y) * (r_des.theta_ddot + abs(K_d.hor.theta) * (r_des.theta_dot - theta_dot) + abs(K_p.hor.theta) * (theta_des - theta));
    M_z = (params.hor.J_zz / params.hor.L_z) * (r_des.psi_ddot + abs(K_d.hor.psi) * (r_des.psi_dot - psi_dot) + abs(K_p.hor.psi) * (psi_des - psi));
    
else 
    
    M_x = (params.ver.J_xx / params.ver.L_x) * (r_des.fi_ddot + abs(K_d.ver.fi) * (r_des.fi_dot - fi_dot) + abs(K_p.ver.fi) * (fi_des - fi));
    M_y = (params.ver.J_yy / params.ver.L_y) * (r_des.theta_ddot + abs(K_d.ver.theta) * (r_des.theta_dot - theta_dot) + abs(K_p.ver.theta) * (theta_des - theta));
    M_z = (params.ver.J_zz / params.ver.L_z) * (r_des.psi_ddot + abs(K_d.ver.psi) * (r_des.psi_dot - psi_dot) + abs(K_p.ver.psi) * (psi_des - psi));
    
end

== matlab function sistem_full/MATLAB Function9 ==
  data: alpha_1 output; alpha_2 output; alpha_3 output; alpha_4 output; F_T input; Y input; w output; M_x input; M_y input; M_z input; x_dot input; params input; alpha_L output; alpha_R output; alpha_H output; alpha_F output; mode input
function [alpha_1, alpha_2, alpha_3, alpha_4, w, alpha_L, alpha_R, alpha_H, alpha_F] = fcn(F_T, Y, M_x, M_y, M_z, x_dot, params, mode)

if mode == 0
    
    alpha_1 = (1 / (4 * params.k_Y)) * (F_T + M_x + M_y + M_z) - 7;
    alpha_2 = (1 / (4 * params.k_Y)) * (F_T + M_x - M_y - M_z);
    alpha_3 = (1 / (4 * params.k_Y)) * (F_T - M_x + M_y - M_z) - 7;
    alpha_4 = (1 / (4 * params.k_Y)) * (F_T - M_x - M_y + M_z);
    
    w = params.w_0;
    alpha_L = -7;
    alpha_R = -7;
    alpha_H = 0;
    alpha_F = 0;
    
elseif mode == 1
    
    alpha_1 = 7.5;
    alpha_2 = 7.5;
    alpha_3 = 7.5;
    alpha_4 = 7.5;

    w = (50000 * F_T + 245100) / 77;

    alpha_L = (500 * M_x + 500 * Y + 102201 * params.S_k * params.rho - 14630 * params.S_k * params.rho * x_dot) / (30 * params.S_k * params.rho * (70 * x_dot - 489));
    alpha_R = - (500 * M_x - 500 * Y - 102201 * params.S_k * params.rho + 14630 * params.S_k * params.rho * x_dot) / (30 * params.S_k * params.rho * (70 * x_dot - 489));
    alpha_H = (125 * M_y) / (3 * params.S_h * params.rho * (70 * x_dot - 489));
    alpha_F = (125 * M_z) / (3 * params.S_f * params.rho * (70 * x_dot - 489));
    
else
    
    alpha_1 = (1 / (4 * params.k_Y)) * (F_T + M_x + M_y + M_z) - 7;
    alpha_2 = (1 / (4 * params.k_Y)) * (F_T + M_x - M_y - M_z);
    alpha_3 = (1 / (4 * params.k_Y)) * (F_T - M_x + M_y - M_z) - 7;
    alpha_4 = (1 / (4 * params.k_Y)) * (F_T - M_x - M_y + M_z);
    
    w = params.w_0;
    alpha_L = -7;
    alpha_R = -7;
    alpha_H = 0;
    alpha_F = 0;
    
end

== matlab function sistem_full/MATLAB Function10 ==
  data: w_L input; F output; w_R input; alpha_1 input; alpha_2 input; alpha_3 input; alpha_4 input; params input
function F = fcn(w_L, w_R, alpha_1, alpha_2, alpha_3, alpha_4, params)
alpha_L = alpha_1 + alpha_2;
alpha_R = alpha_3 + alpha_4;

C_Y_L = 0.1545 * (alpha_L + 7);
C_Y_R = 0.1545 * (alpha_R + 7);

F = (3/2) * params.rho * params.S_l * (C_Y_L * w_L^2 + C_Y_R * w_R^2);

== matlab function sistem_full/MATLAB Function11 ==
  data: w_L input; M_x output; w_R input; alpha_1 input; alpha_2 input; alpha_3 input; alpha_4 input; params input; M_y output; M_z output
function [M_x, M_y, M_z] = fcn(w_L, w_R, alpha_1, alpha_2, alpha_3, alpha_4, params)

%alpha_1 = alpha_1 * pi / 180;
%alpha_2 = alpha_2 * pi / 180;
%alpha_3 = alpha_3 * pi / 180;
%alpha_4 = alpha_4 * pi / 180;

%M_x = params.k_F * (w_L^2 * (alpha_1 + alpha_2) - w_R^2 * (alpha_3 + alpha_4));
%M_y = params.k_F * (w_L^2 * (alpha_1 - alpha_2) + w_R^2 * (alpha_3 - alpha_4));
%M_z = params.k_F * (w_L^2 * (alpha_1 - alpha_2) - w_R^2 * (alpha_3 - alpha_4));

M_x = (3/2) * params.rho * params.S_l * (0.1545 * ((alpha_1 + alpha_2) + 7) * w_L^2 - 0.1545 * ((alpha_3 + alpha_4) + 7) * w_R^2);
M_y = (3/2) * params.rho * params.S_l * (0.1545 * ((alpha_1 - alpha_2) + 7) * w_L^2 + 0.1545 * ((alpha_3 - alpha_4) + 7) * w_R^2);
M_z = (3/2) * params.rho * params.S_l * (0.1545 * ((alpha_1 - alpha_2) + 7) * w_L^2 - 0.1545 * ((alpha_3 - alpha_4) + 7) * w_R^2);

== matlab function sistem_full/MATLAB Function12 ==
  data: F input; F_x output; fi input; theta input; psi input; F_y output; F_z output
function [F_x, F_y, F_z] = fcn(F, fi, theta, psi)

F_x = F * (cos(psi) * theta + fi * sin(psi));
F_y = F * (sin(psi) * theta - cos(psi) * fi);
F_z = F;

== matlab function sistem_full/MATLAB Function13 ==
  data: F_x input; x_ddot output; F_y input; F_z input; params input; y_ddot output; z_ddot output
function [x_ddot, y_ddot, z_ddot] = fcn(F_x, F_y, F_z, params)

x_ddot = (1 / params.m) * F_x;
y_ddot = (1 / params.m) * F_y;
z_ddot = (1 / params.m) * (F_z - params.m * params.g);

== matlab function sistem_full/MATLAB Function5 ==
  data: t input; coeff output; r_0 input; r_end input
function coeff  = calculation_coefficients(t, r_0, r_end)

x_0 = r_0;
x_dot_0 = 0;
x_ddot_0 = 0;

x_des = r_end;
x_dot_des = 0;
x_ddot_des = 0;

waypoints = [x_0    x_dot_0     x_ddot_0;
             x_des  x_dot_des   x_ddot_des]';
t = [0 t];

time_size = size(t);
n = 0;
%T = linspace(0, time_size(2) - 1, point(2));


border_conditions_sigm = reshape(waypoints(:, n + 1 : n + 2),1,[]);
%disp(border_conditions_sigm)

coeff = zeros(6, 1);

parameters = [1 * (t(n + 1) ^ 5), 1 * (t(n + 1) ^ 4), 1 * (t(n + 1) ^ 3), 1 * (t(n + 1) ^ 2), 1 * (t(n + 1) ^ 1), 1 * (t(n + 1) ^ 0);
              5 * (t(n + 1) ^ 4), 4 * (t(n + 1) ^ 3), 3 * (t(n + 1) ^ 2), 2 * (t(n + 1) ^ 1), 1 * (t(n + 1) ^ 0), 0 * (t(n + 1) ^ 0);
              20 * (t(n + 1) ^ 3), 12 * (t(n + 1) ^ 2), 6 * (t(n + 1) ^ 1), 2 * (t(n + 1) ^ 0), 0 * (t(n + 1) ^ 0), 0 * (t(n + 1) ^ 0);
              1 * (t(n + 2) ^ 5), 1 * (t(n + 2) ^ 4), 1 * (t(n + 2) ^ 3), 1 * (t(n + 2) ^ 2), 1 * (t(n + 2) ^ 1), 1 * (t(n + 2) ^ 0);
              5 * (t(n + 2) ^ 4), 4 * (t(n + 2) ^ 3), 3 * (t(n + 2) ^ 2), 2 * (t(n + 2) ^ 1), 1 * (t(n + 2) ^ 0), 0 * (t(n + 2) ^ 0);
              20 * (t(n + 2) ^ 3), 12 * (t(n + 2) ^ 2), 6 * (t(n + 2) ^ 1), 2 * (t(n + 2) ^ 0), 0 * (t(n + 2) ^ 0), 0 * (t(n + 2) ^ 0)];

coeff = inv(parameters) * border_conditions_sigm';

== stateflow chart sistem_full/Chart1 ==
  state Vertical_flight
    mode = 0
    sigma = 0
  state Horizontal_flight
    mode = 1
    sigma = 90
  (default) -> Vertical_flight
  Horizontal_flight -> Vertical_flight : [x_dot_des < 14.1]
  Vertical_flight -> Horizontal_flight : [x_dot_des > 14.1]
  data: mode output; x_dot_des input; sigma output

== matlab function sistem_full/MATLAB Function14 ==
  data: w_L input; F output; w_R input; params input
function F  = fcn(w_L, w_R, params)
F = params.k_F * (w_L^2 + w_R^2);

== matlab function sistem_full/MATLAB Function15 ==
  data: x_dot input; alpha_L input; alpha_R input; params input; Y output
function Y = fcn(x_dot, alpha_L, alpha_R, params)

C_y_L = 0.1029 + 0.1498 * (alpha_L + 6.3236);
C_y_R = 0.1029 + 0.1498 * (alpha_R + 6.3236);
v = 196.4002 + 28.0286 * (x_dot - 14.0143);

Y = (1 / 2) * params.rho * v * params.S_k * (C_y_L + C_y_R);

== matlab function sistem_full/MATLAB Function16 ==
  data: x_dot input; M_x output; alpha_L input; alpha_R input; alpha_H input; alpha_F input; M_y output; M_z output; params input
function [M_x, M_y, M_z] = fcn(x_dot, alpha_L, alpha_R, alpha_H, alpha_F, params)

C_y_L = 0.1029 + 0.1498 * (alpha_L + 6.3236);
C_y_R = 0.1029 + 0.1498 * (alpha_R + 6.3236);
C_y_H = 0.12 * alpha_H;
C_y_F = 0.12 * alpha_F;
v = 196.4002 + 28.0286 * (x_dot - 14.0143);


M_x = (1 / 2) * params.rho * v * params.S_k * (C_y_L - C_y_R);
M_y = C_y_H * (1 / 2) * params.rho * v * params.S_h;
M_z = C_y_F * (1 / 2) * params.rho * v * params.S_f;

== matlab function sistem_full/MATLAB Function17 ==
  data: F input; F_x output; fi input; theta input; psi input; F_y output; F_z output
function [F_x, F_y, F_z] = fcn(F, fi, theta, psi)

F_x = F;
F_y = F * (cos(fi) * psi + sin(fi) * theta);
F_z = F * (sin(fi) * psi - cos(fi) * theta);

== matlab function sistem_full/MATLAB Function1 ==
  data: t input; coeff output; r_0 input; r_end input
function coeff  = calculation_coefficients(t, r_0, r_end)

x_0 = r_0;
x_dot_0 = 0;
x_ddot_0 = 0;

x_des = r_end;
x_dot_des = 0;
x_ddot_des = 0;

waypoints = [x_0    x_dot_0     x_ddot_0;
             x_des  x_dot_des   x_ddot_des]';
t = [0 t];

time_size = size(t);
n = 0;
%T = linspace(0, time_size(2) - 1, point(2));


border_conditions_sigm = reshape(waypoints(:, n + 1 : n + 2),1,[]);
%disp(border_conditions_sigm)

coeff = zeros(6, 1);

parameters = [1 * (t(n + 1) ^ 5), 1 * (t(n + 1) ^ 4), 1 * (t(n + 1) ^ 3), 1 * (t(n + 1) ^ 2), 1 * (t(n + 1) ^ 1), 1 * (t(n + 1) ^ 0);
              5 * (t(n + 1) ^ 4), 4 * (t(n + 1) ^ 3), 3 * (t(n + 1) ^ 2), 2 * (t(n + 1) ^ 1), 1 * (t(n + 1) ^ 0), 0 * (t(n + 1) ^ 0);
              20 * (t(n + 1) ^ 3), 12 * (t(n + 1) ^ 2), 6 * (t(n + 1) ^ 1), 2 * (t(n + 1) ^ 0), 0 * (t(n + 1) ^ 0), 0 * (t(n + 1) ^ 0);
              1 * (t(n + 2) ^ 5), 1 * (t(n + 2) ^ 4), 1 * (t(n + 2) ^ 3), 1 * (t(n + 2) ^ 2), 1 * (t(n + 2) ^ 1), 1 * (t(n + 2) ^ 0);
              5 * (t(n + 2) ^ 4), 4 * (t(n + 2) ^ 3), 3 * (t(n + 2) ^ 2), 2 * (t(n + 2) ^ 1), 1 * (t(n + 2) ^ 0), 0 * (t(n + 2) ^ 0);
              20 * (t(n + 2) ^ 3), 12 * (t(n + 2) ^ 2), 6 * (t(n + 2) ^ 1), 2 * (t(n + 2) ^ 0), 0 * (t(n + 2) ^ 0), 0 * (t(n + 2) ^ 0)];

coeff = inv(parameters) * border_conditions_sigm';

== matlab function sistem_full/MATLAB Function18 ==
  data: coeff input; pos output; clock input; vel output; acc output
function [pos, vel, acc] = trajectories_calculation(coeff, clock)

T_p = [clock^5      clock^4     clock^3     clock^2     clock   1]';
T_v = [5*clock^4    4*clock^3   3*clock^2   2*clock     1       0]';
T_a = [20*clock^3   12*clock^2  6*clock     2           0       0]';

pos = sum(coeff.*T_p);
vel = sum(coeff.*T_v);
acc = sum(coeff.*T_a);
